simulink model "gm_GammaCorrectionHDLExample"  (R2017a)
settings: Solver=FixedStepDiscrete  StartTime=0.0  StopTime=402*324*10  RelTol=1e-3
PreLoadFcn:
  | gammaValue=2.2;
undefined symbols (not defined in the file or in its folder): gray
libraries: visionconversions x2, visionhdlio x2, visionstatistics x2, visionhdlmisc x1, visionhdlconversions x1, dspvision x1
settings Model: SimulationMode=accelerator  Creator=The MathWorks, Inc.  LastModifiedBy=dilin
settings DataIOCC: LimitDataPoints=on  SaveFormat=Structure  SaveTime=off
settings OptimizationCC: BlockReduction=off  ConditionallyExecuteInputs=off  DefaultParameterBehavior=Inlined  LifeSpan=inf
settings DebuggingCC: AlgebraicLoopMsg=error  UnderspecifiedInitializationDetection=Classic  MergeDetectMultiDrivingBlocksExec=none  SolverPrmCheckMsg=warning  InheritedTsInSrcMsg=none  ParameterPrecisionLossMsg=none  AllowSymbolicDim=off  SFUnexpectedBacktrackingDiag=warning  SFNoUnconditionalDefaultTransitionDiag=warning  SFExecutionAtInitializationDiag=none
settings HardwareCC: ProdBitPerPointer=32  ProdBitPerSizeT=32  ProdBitPerPtrDiffT=32  ProdLargestAtomicFloat=None  ProdIntDivRoundTo=Undefined  ProdEndianess=Unspecified  ProdWordSize=32  ProdHWDeviceType=ASIC/FPGA->ASIC/FPGA  ProdEqTarget=off
settings ModelReferenceCC: PropagateSignalLabelsOutOfModel=off
settings GRTTargetCC: TargetLangStandard=C89/C90 (ANSI)  GeneratePreprocessorConditionals=Disable all
settings ConfigComp: CovMetricSettings=dw  CovHtmlReporting=on  CovSaveCumulativeToWorkspaceVar=on  CovSaveSingleToWorkspaceVar=on  CovExternalEMLEnable=off  CovSFcnEnable=off

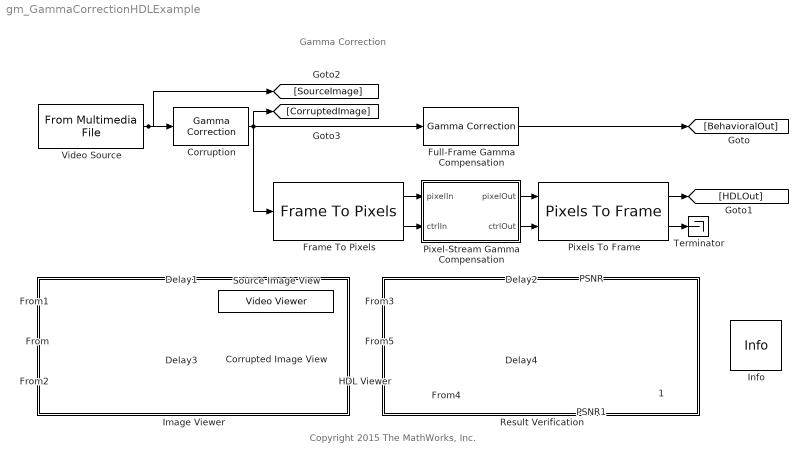
== system gm_GammaCorrectionHDLExample ==
  note: Gamma Correction
  note: Copyright 2015 The MathWorks, Inc.
  " " : Display
  " 1" : Display
  Corrupted Image View : VideoViewer  colormapValue=gray(256)  FigPos=[372 383 331 268]
  Corruption : visionconversions/Gamma Correction  operation=De-gamma  gamma=gammaValue  linearSegment=off  breakPoint=0.018
      settings: SourceProductName=Computer Vision System Toolbox  SourceProductBaseCode=VP
  Delay{1..4} (4 alike) : Delay  DelayLength=1  InitialCondition=0
  Frame To Pixels : visionhdlio/Frame To Pixels  NumComponents=1  VideoFormat=240p  ActivePixelsPerLine=32  ActiveVideoLines=18  TotalPixelsPerLine=42  TotalVideoLines=28  StartingActiveLine=6  FrontPorch=5  SampleTime=0
      settings: SourceProductName=Vision HDL Toolbox  SourceProductBaseCode=VT
  Full-Frame Gamma Compensation : visionconversions/Gamma Correction  operation=Gamma  gamma=gammaValue  linearSegment=off  breakPoint=0.018
      settings: SourceProductName=Computer Vision System Toolbox  SourceProductBaseCode=VP
  HDL Viewer : VideoViewer  colormapValue=gray(256)  FigPos=[685 386 351 280]
  Image Viewer : Subsystem
      mask Display: disp('')
  Info : visionhdlmisc/Info  SystemSampleTime=-1
      settings: SourceProductName=Vision HDL Toolbox  SourceProductBaseCode=VT
  PSNR : visionstatistics/PSNR
      settings: SourceProductName=Computer Vision System Toolbox  SourceProductBaseCode=VP
  PSNR1 : visionstatistics/PSNR
      settings: SourceProductName=Computer Vision System Toolbox  SourceProductBaseCode=VP
  Pixel-Stream Gamma Compensation : Subsystem  TreatAsAtomicUnit=on
  Pixels To Frame : visionhdlio/Pixels To Frame  NumComponents=1  VideoFormat=240p  ActivePixelsPerLine=32  ActiveVideoLines=18  TotalPixelsPerLine=42  TotalVideoLines=28
      settings: SourceProductName=Vision HDL Toolbox  SourceProductBaseCode=VT
  Result Verification : Subsystem
      mask Display: disp('')
  Source Image View : VideoViewer  colormapValue=gray(256)  FigPos=[36 385 350 276]
  Terminator : Terminator
  Video Source : dspvision/From Multimedia File  inputFilename=rhinos.avi  loop=on  numPlays=inf  outputStreams=Video only  videoDataType=uint8  audioDataType=int16  inheritSampleTime=off  userDefinedSampleTime=402*324  noAudioOutput=off  isIntensityVideo=off  fourcc=Intensity  colorVideoFormat=One multidimensional signal  outputEOF=off  dataOrg=Column-major  audioFrameSize=1024  computeAudioFrameSize=off  outSamplingMode=Sample based
      settings: SourceProductBaseCode=VP
  wires:
  [BehavioralOut] -> Delay4/1
  [SourceImage] -> Delay2/1
  [HDLOut] -> PSNR1/2
  Delay4/1 -> PSNR/2, PSNR1/1
  [HDLOut] -> HDL Viewer/1
  [SourceImage] -> Delay1/1
  [CorruptedImage] -> Delay3/1
  Delay3/1 -> Corrupted Image View/1
  Delay1/1 -> Source Image View/1
  Delay2/1 -> PSNR/1
  PSNR/1 -> " "/1
  PSNR1/1 -> " 1"/1
  Full-Frame Gamma Compensation/1 -> [BehavioralOut]
  Corruption/1 -> [CorruptedImage], Full-Frame Gamma Compensation/1, Frame To Pixels/1
  Video Source/1 -> Corruption/1, [SourceImage]
  Pixels To Frame/1 -> [HDLOut]
  Pixel-Stream Gamma Compensation/2(ctrlOut) -> Pixels To Frame/2
  Pixel-Stream Gamma Compensation/1(pixelOut) -> Pixels To Frame/1
  Frame To Pixels/2 -> Pixel-Stream Gamma Compensation/2(ctrlIn)
  Frame To Pixels/1 -> Pixel-Stream Gamma Compensation/1(pixelIn)
  Pixels To Frame/2 -> Terminator/1

== system gm_GammaCorrectionHDLExample/Image Viewer ==

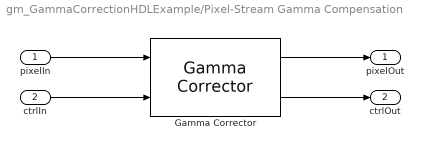
== system gm_GammaCorrectionHDLExample/Pixel-Stream Gamma Compensation ==
  pixelIn : Inport
  ctrlIn : Inport  Port=2
  Gamma Corrector : visionhdlconversions/Gamma Corrector  Correction=Gamma  Gamma=gammaValue  LinearSegment=off  BreakPoint=0.018  SimulateUsing=Code generation
      settings: SourceProductName=Vision HDL Toolbox  SourceProductBaseCode=VT
  pixelOut : Outport
  ctrlOut : Outport  Port=2
  wires:
  Gamma Corrector/2 -> ctrlOut/1
  Gamma Corrector/1 -> pixelOut/1
  ctrlIn/1 -> Gamma Corrector/2
  pixelIn/1 -> Gamma Corrector/1

== system gm_GammaCorrectionHDLExample/Result Verification ==
